simulink model "VTOLDynamics"  (R2024b)
settings: Solver=ode23t  StartTime=0.0  StopTime=10.0  FixedStep=0.001  RelTol=1e-3
undefined symbols (not defined in the file): const, contact, env, F, Flap_Activate, iniRoll, initPitch, iniYaw, Light, Limit, MIL, motorctrl, tiltIni, uavParam, uavParams, vIni, xGround, yGround, zGround
libraries: matrix_library x8, slpidlib x4, robotcorelib x4, aerolibasang x2, aerolibwind2 x2, sharedtransform x2, shared6dof x1, aerolibadyn x1, sharedutil x1, Uav_Electrical_lib x1, aerolibatmos2 x1
(part 3 of 3)

== system VTOLDynamics/Force and Moments/Aerodynamic Forces/Compute Body Frame Forces and Moments/Wind frame F& M/Lateral Channel/CY/roll factors ==
  p,q,r : Inport
  Airspeed : Inport  Port=2
  Constant : Constant  Value=uavParams.aero.CYp
      settings: AttributesFormatString=%<Value>
  Constant1 : Constant  Value=uavParams.aero.CYr
      settings: AttributesFormatString=%<Value>
  Product : Product  SaturateOnIntegerOverflow=on  OutDataTypeStr=Inherit: Same as first input
  Product1 : Product  SaturateOnIntegerOverflow=on  OutDataTypeStr=Inherit: Same as first input
  Selector : Selector  InputPortWidth=3  IndexOptions=Index vector (dialog)  Indices=[1]  OutputSizes=1
  Selector1 : Selector  InputPortWidth=3  IndexOptions=Index vector (dialog)  Indices=[3]  OutputSizes=1
  Subsystem : Subsystem
  roll rate fact : Subsystem
  CSp : Outport  VectorParamsAs1DForOutWhenUnconnected=off
  CSr : Outport  Port=2  VectorParamsAs1DForOutWhenUnconnected=off
  wires:
  Selector1/1 -> Subsystem/1(r)
  p,q,r/1 -> Selector1/1, Selector/1
  Selector/1 -> roll rate fact/1(p)
  Airspeed/1 -> Subsystem/2(Airspeed), roll rate fact/2(Airspeed)
  Subsystem/1(Yaw Rate Fac) -> Product1/2
  roll rate fact/1(Roll Rate Fac) -> Product/2
  Product1/1 -> CSr/1
  Product/1 -> CSp/1
  Constant/1 -> Product/1
  Constant1/1 -> Product1/1

== system VTOLDynamics/Force and Moments/Aerodynamic Forces/Compute Body Frame Forces and Moments/Wind frame F& M/Lateral Channel/Cl/roll factors ==
  p,q,r : Inport
  Airspeed : Inport  Port=2
  Constant : Constant  Value=uavParams.aero.Clp
      settings: AttributesFormatString=%<Value>
  Constant1 : Constant  Value=uavParams.aero.Clr
      settings: AttributesFormatString=%<Value>
  Product : Product  SaturateOnIntegerOverflow=on  OutDataTypeStr=Inherit: Same as first input
  Product1 : Product  SaturateOnIntegerOverflow=on  OutDataTypeStr=Inherit: Same as first input
  Selector : Selector  InputPortWidth=3  IndexOptions=Index vector (dialog)  Indices=[1]  OutputSizes=1
  Selector1 : Selector  InputPortWidth=3  IndexOptions=Index vector (dialog)  Indices=[3]  OutputSizes=1
  roll rate fact : Subsystem
  yaw rate fact : Subsystem
  Clp : Outport  VectorParamsAs1DForOutWhenUnconnected=off
  Clr : Outport  Port=2  VectorParamsAs1DForOutWhenUnconnected=off
  wires:
  Selector1/1 -> yaw rate fact/1(r)
  p,q,r/1 -> Selector1/1, Selector/1
  Selector/1 -> roll rate fact/1(p)
  Airspeed/1 -> roll rate fact/2(Airspeed), yaw rate fact/2(Airspeed)
  yaw rate fact/1(Yaw Rate Fac) -> Product1/2
  Constant1/1 -> Product1/1
  roll rate fact/1(Roll Rate Fac) -> Product/2
  Constant/1 -> Product/1
  Product1/1 -> Clr/1
  Product/1 -> Clp/1

== system VTOLDynamics/Force and Moments/Aerodynamic Forces/Compute Body Frame Forces and Moments/Wind frame F& M/Lateral Channel/Cn/yaw factors ==
  p,q,r : Inport
  Airspeed : Inport  Port=2
  Constant : Constant  Value=uavParams.aero.Cnp
      settings: AttributesFormatString=%<Value>
  Constant1 : Constant  Value=uavParams.aero.Cnr
      settings: AttributesFormatString=%<Value>
  Product : Product  SaturateOnIntegerOverflow=on  OutDataTypeStr=Inherit: Same as first input
  Product1 : Product  SaturateOnIntegerOverflow=on  OutDataTypeStr=Inherit: Same as first input
  Selector : Selector  InputPortWidth=3  IndexOptions=Index vector (dialog)  Indices=[3]  OutputSizes=1
  Selector1 : Selector  InputPortWidth=3  IndexOptions=Index vector (dialog)  Indices=[1]  OutputSizes=1
  roll rate fact : Subsystem
  yaw rate fact1 : Subsystem
  Cnp : Outport  VectorParamsAs1DForOutWhenUnconnected=off
  Cnr : Outport  Port=2  VectorParamsAs1DForOutWhenUnconnected=off
  wires:
  Airspeed/1 -> yaw rate fact1/2(Airspeed), roll rate fact/2(Airspeed)
  Selector/1 -> yaw rate fact1/1(r)
  p,q,r/1 -> Selector1/1, Selector/1
  Selector1/1 -> roll rate fact/1(p)
  roll rate fact/1(Roll Rate Fac) -> Product/2
  Constant/1 -> Product/1
  yaw rate fact1/1(Yaw Rate Fac) -> Product1/2
  Constant1/1 -> Product1/1
  Product1/1 -> Cnr/1
  Product/1 -> Cnp/1

== system VTOLDynamics/Force and Moments/Aerodynamic Forces/Compute Body Frame Forces and Moments/Wind frame F& M/Longitudinal Channel/CL/Lift due to pitch rate ==
  p,q,r : Inport
  Airspeed : Inport  Port=2
  Constant : Constant  Value=uavParams.aero.CLq
      settings: AttributesFormatString=%<Value>
  Product : Product  SaturateOnIntegerOverflow=on  OutDataTypeStr=Inherit: Same as first input
  Selector : Selector  InputPortWidth=3  IndexOptions=Index vector (dialog)  Indices=[2]  OutputSizes=1
  pitch rate factor : Subsystem
  CLq : Outport  VectorParamsAs1DForOutWhenUnconnected=off
  wires:
  Airspeed/1 -> pitch rate factor/2(Airspeed)
  Selector/1 -> pitch rate factor/1(q)
  p,q,r/1 -> Selector/1
  Product/1 -> CLq/1
  pitch rate factor/1(Pitch Rate Fac) -> Product/2
  Constant/1 -> Product/1

== system VTOLDynamics/Force and Moments/Aerodynamic Forces/Compute Body Frame Forces and Moments/Wind frame F& M/Longitudinal Channel/Cm/Lift due to pitch rate ==
  p,q,r : Inport
  Airspeed : Inport  Port=2
  Constant : Constant  Value=uavParams.aero.Cmq
      settings: AttributesFormatString=%<Value>
  Product : Product  SaturateOnIntegerOverflow=on  OutDataTypeStr=Inherit: Same as first input
  Selector : Selector  InputPortWidth=3  IndexOptions=Index vector (dialog)  Indices=[2]  OutputSizes=1
  pitch rate factor : Subsystem
  Cmq : Outport  VectorParamsAs1DForOutWhenUnconnected=off
  wires:
  Airspeed/1 -> pitch rate factor/2(Airspeed)
  Selector/1 -> pitch rate factor/1(q)
  p,q,r/1 -> Selector/1
  Product/1 -> Cmq/1
  pitch rate factor/1(Pitch Rate Fac) -> Product/2
  Constant/1 -> Product/1

== system VTOLDynamics/Force and Moments/Aerodynamic Forces/Compute Body Frame Forces and Moments/Wind frame F& M_original/Lateral Channel/CY/roll factors ==
  p,q,r : Inport
  Airspeed : Inport  Port=2
  Constant : Constant  Value=uavParam.aero.CYp
      settings: AttributesFormatString=%<Value>
  Constant1 : Constant  Value=uavParam.aero.CYr
      settings: AttributesFormatString=%<Value>
  Get p : Selector  InputPortWidth=3  IndexOptions=Index vector (dialog)  Indices=1  OutputSizes=[(-2)]
  Get r : Selector  InputPortWidth=3  IndexOptions=Index vector (dialog)  Indices=3  OutputSizes=[(-2)]
  Product : Product  SaturateOnIntegerOverflow=on  OutDataTypeStr=Inherit: Same as first input
  Product1 : Product  SaturateOnIntegerOverflow=on  OutDataTypeStr=Inherit: Same as first input
  Subsystem : Subsystem
  roll rate fact : Subsystem
  CYp : Outport  VectorParamsAs1DForOutWhenUnconnected=off
  CYr : Outport  Port=2  VectorParamsAs1DForOutWhenUnconnected=off
  wires:
  Get r/1 -> Subsystem/1(r)
  p,q,r/1 -> Get r/1, Get p/1
  Get p/1 -> roll rate fact/1(p)
  Airspeed/1 -> Subsystem/2(Airspeed), roll rate fact/2(Airspeed)
  Subsystem/1(Yaw Rate Fac) -> Product1/2
  Constant1/1 -> Product1/1
  roll rate fact/1(Roll Rate Fac) -> Product/2
  Constant/1 -> Product/1
  Product1/1 -> CYr/1
  Product/1 -> CYp/1

== system VTOLDynamics/Force and Moments/Aerodynamic Forces/Compute Body Frame Forces and Moments/Wind frame F& M_original/Lateral Channel/Cl/roll factors ==
  p,q,r : Inport
  Airspeed : Inport  Port=2
  Constant : Constant  Value=uavParam.aero.Clp
      settings: AttributesFormatString=%<Value>
  Constant1 : Constant  Value=uavParam.aero.Clr
      settings: AttributesFormatString=%<Value>
  Get p : Selector  InputPortWidth=3  IndexOptions=Index vector (dialog)  Indices=1  OutputSizes=[(-2)]
  Get r : Selector  InputPortWidth=3  IndexOptions=Index vector (dialog)  Indices=3  OutputSizes=[(-2)]
  Product : Product  SaturateOnIntegerOverflow=on  OutDataTypeStr=Inherit: Same as first input
  Product1 : Product  SaturateOnIntegerOverflow=on  OutDataTypeStr=Inherit: Same as first input
  roll rate fact : Subsystem
  yaw rate fact : Subsystem
  Clp : Outport  VectorParamsAs1DForOutWhenUnconnected=off
  Clr : Outport  Port=2  VectorParamsAs1DForOutWhenUnconnected=off
  wires:
  Get r/1 -> yaw rate fact/1(r)
  p,q,r/1 -> Get r/1, Get p/1
  Get p/1 -> roll rate fact/1(p)
  Airspeed/1 -> yaw rate fact/2(Airspeed), roll rate fact/2(Airspeed)
  yaw rate fact/1(Yaw Rate Fac) -> Product1/2
  Constant1/1 -> Product1/1
  roll rate fact/1(Roll Rate Fac) -> Product/2
  Constant/1 -> Product/1
  Product1/1 -> Clr/1
  Product/1 -> Clp/1

== system VTOLDynamics/Force and Moments/Aerodynamic Forces/Compute Body Frame Forces and Moments/Wind frame F& M_original/Lateral Channel/Cn/yaw factors ==
  p,q,r : Inport
  Airspeed : Inport  Port=2
  Constant : Constant  Value=uavParam.aero.Cnp
      settings: AttributesFormatString=%<Value>
  Constant1 : Constant  Value=uavParam.aero.Cnr
      settings: AttributesFormatString=%<Value>
  Get p : Selector  InputPortWidth=3  IndexOptions=Index vector (dialog)  Indices=1  OutputSizes=[(-2)]
  Get r : Selector  InputPortWidth=3  IndexOptions=Index vector (dialog)  Indices=3  OutputSizes=[(-2)]
  Product : Product  SaturateOnIntegerOverflow=on  OutDataTypeStr=Inherit: Same as first input
  Product1 : Product  SaturateOnIntegerOverflow=on  OutDataTypeStr=Inherit: Same as first input
  roll rate fact : Subsystem
  yaw rate fact1 : Subsystem
  Cnp : Outport  VectorParamsAs1DForOutWhenUnconnected=off
  Cnr : Outport  Port=2  VectorParamsAs1DForOutWhenUnconnected=off
  wires:
  Airspeed/1 -> yaw rate fact1/2(Airspeed), roll rate fact/2(Airspeed)
  Get r/1 -> yaw rate fact1/1(r)
  p,q,r/1 -> Get r/1, Get p/1
  Get p/1 -> roll rate fact/1(p)
  roll rate fact/1(Roll Rate Fac) -> Product/2
  Constant/1 -> Product/1
  yaw rate fact1/1(Yaw Rate Fac) -> Product1/2
  Constant1/1 -> Product1/1
  Product1/1 -> Cnr/1
  Product/1 -> Cnp/1

== system VTOLDynamics/Force and Moments/Aerodynamic Forces/Compute Body Frame Forces and Moments/Wind frame F& M_original/Longitudinal Channel/CL/Lift due to pitch rate ==
  p,q,r : Inport
  Airspeed : Inport  Port=2
  Constant : Constant  Value=uavParam.aero.CLq
      settings: AttributesFormatString=%<Value>
  Get q : Selector  InputPortWidth=3  IndexOptions=Index vector (dialog)  Indices=2  OutputSizes=[(-2)]
  Product : Product  SaturateOnIntegerOverflow=on  OutDataTypeStr=Inherit: Same as first input
  pitch rate factor : Subsystem
  CLq : Outport  VectorParamsAs1DForOutWhenUnconnected=off
  wires:
  Airspeed/1 -> pitch rate factor/2(Airspeed)
  Get q/1 -> pitch rate factor/1(q)
  p,q,r/1 -> Get q/1
  Product/1 -> CLq/1
  pitch rate factor/1(Pitch Rate Fac) -> Product/2
  Constant/1 -> Product/1

== system VTOLDynamics/Force and Moments/Aerodynamic Forces/Compute Body Frame Forces and Moments/Wind frame F& M_original/Longitudinal Channel/Cm/Lift due to pitch rate ==
  p,q,r : Inport
  Airspeed : Inport  Port=2
  Constant : Constant  Value=uavParam.aero.Cmq
      settings: AttributesFormatString=%<Value>
  Get q : Selector  InputPortWidth=3  IndexOptions=Index vector (dialog)  Indices=2  OutputSizes=[(-2)]
  Product : Product  SaturateOnIntegerOverflow=on  OutDataTypeStr=Inherit: Same as first input
  pitch rate factor : Subsystem
  Cmq : Outport  VectorParamsAs1DForOutWhenUnconnected=off
  wires:
  Airspeed/1 -> pitch rate factor/2(Airspeed)
  Get q/1 -> pitch rate factor/1(q)
  p,q,r/1 -> Get q/1
  Product/1 -> Cmq/1
  pitch rate factor/1(Pitch Rate Fac) -> Product/2
  Constant/1 -> Product/1

== system VTOLDynamics/Force and Moments/Aerodynamic Forces/Compute Body Frame Forces and Moments/Wind frame F& M/Lateral Channel/CY/roll factors/Subsystem ==
  r : Inport
  Airspeed : Inport  Port=2
  Cmq4 : Constant  Value=uavParams.geom.b
      settings: AttributesFormatString=%<Value>
  Gain : Gain  Gain=2
  Product1 : Product  Inputs=**/  SaturateOnIntegerOverflow=on  OutDataTypeStr=Inherit: Same as first input
  Saturation : Saturate  UpperLimit=inf  LowerLimit=0.1
      settings: AttributesFormatString="[%<LowerLimit>  %<UpperLimit>]"
  Yaw Rate Fac : Outport  VectorParamsAs1DForOutWhenUnconnected=off
  wires:
  Saturation/1 -> Gain/1
  Airspeed/1 -> Saturation/1
  Gain/1 -> Product1/3
  Product1/1 -> Yaw Rate Fac/1
  r/1 -> Product1/1
  Cmq4/1 -> Product1/2

== system VTOLDynamics/Force and Moments/Aerodynamic Forces/Compute Body Frame Forces and Moments/Wind frame F& M/Lateral Channel/CY/roll factors/roll rate fact ==
  p : Inport
  Airspeed : Inport  Port=2
  Cmq2 : Constant  Value=uavParams.geom.b
      settings: AttributesFormatString=%<Value>
  Gain : Gain  Gain=2
  Product : Product  Inputs=**/  SaturateOnIntegerOverflow=on  OutDataTypeStr=Inherit: Same as first input
  Saturation : Saturate  UpperLimit=inf  LowerLimit=0.1
      settings: AttributesFormatString="[%<LowerLimit>  %<UpperLimit>]"
  Roll Rate Fac : Outport  VectorParamsAs1DForOutWhenUnconnected=off
  wires:
  Airspeed/1 -> Saturation/1
  p/1 -> Product/1
  Product/1 -> Roll Rate Fac/1
  Saturation/1 -> Gain/1
  Cmq2/1 -> Product/2
  Gain/1 -> Product/3

== system VTOLDynamics/Force and Moments/Aerodynamic Forces/Compute Body Frame Forces and Moments/Wind frame F& M/Lateral Channel/Cl/roll factors/roll rate fact ==
  p : Inport
  Airspeed : Inport  Port=2
  Cmq2 : Constant  Value=uavParams.geom.b
      settings: AttributesFormatString=%<Value>
  Gain : Gain  Gain=2
  Product : Product  Inputs=**/  SaturateOnIntegerOverflow=on  OutDataTypeStr=Inherit: Same as first input
  Saturation : Saturate  UpperLimit=inf  LowerLimit=0.1
      settings: AttributesFormatString="[%<LowerLimit>  %<UpperLimit>]"
  Roll Rate Fac : Outport  VectorParamsAs1DForOutWhenUnconnected=off
  wires:
  Airspeed/1 -> Saturation/1
  p/1 -> Product/1
  Product/1 -> Roll Rate Fac/1
  Cmq2/1 -> Product/2
  Saturation/1 -> Gain/1
  Gain/1 -> Product/3

== system VTOLDynamics/Force and Moments/Aerodynamic Forces/Compute Body Frame Forces and Moments/Wind frame F& M/Lateral Channel/Cl/roll factors/yaw rate fact ==
  r : Inport
  Airspeed : Inport  Port=2
  Cmq4 : Constant  Value=uavParams.geom.b
      settings: AttributesFormatString=%<Value>
  Gain : Gain  Gain=2
  Product1 : Product  Inputs=**/  SaturateOnIntegerOverflow=on  OutDataTypeStr=Inherit: Same as first input
  Saturation : Saturate  UpperLimit=inf  LowerLimit=0.1
      settings: AttributesFormatString="[%<LowerLimit>  %<UpperLimit>]"
  Yaw Rate Fac : Outport
  wires:
  Airspeed/1 -> Saturation/1
  Saturation/1 -> Gain/1
  r/1 -> Product1/1
  Product1/1 -> Yaw Rate Fac/1
  Cmq4/1 -> Product1/2
  Gain/1 -> Product1/3

== system VTOLDynamics/Force and Moments/Aerodynamic Forces/Compute Body Frame Forces and Moments/Wind frame F& M/Lateral Channel/Cn/yaw factors/roll rate fact ==
  p : Inport
  Airspeed : Inport  Port=2
  Cmq2 : Constant  Value=uavParams.geom.b
      settings: AttributesFormatString=%<Value>
  Gain : Gain  Gain=2
  Product : Product  Inputs=**/  SaturateOnIntegerOverflow=on  OutDataTypeStr=Inherit: Same as first input
  Saturation : Saturate  UpperLimit=inf  LowerLimit=0.1
      settings: AttributesFormatString="[%<LowerLimit>  %<UpperLimit>]"
  Roll Rate Fac : Outport  VectorParamsAs1DForOutWhenUnconnected=off
  wires:
  Saturation/1 -> Gain/1
  Airspeed/1 -> Saturation/1
  p/1 -> Product/1
  Product/1 -> Roll Rate Fac/1
  Gain/1 -> Product/3
  Cmq2/1 -> Product/2

== system VTOLDynamics/Force and Moments/Aerodynamic Forces/Compute Body Frame Forces and Moments/Wind frame F& M/Lateral Channel/Cn/yaw factors/yaw rate fact1 ==
  r : Inport
  Airspeed : Inport  Port=2
  Cmq4 : Constant  Value=uavParams.geom.b
      settings: AttributesFormatString=%<Value>
  Gain : Gain  Gain=2
  Product1 : Product  Inputs=**/  SaturateOnIntegerOverflow=on  OutDataTypeStr=Inherit: Same as first input
  Saturation : Saturate  UpperLimit=inf  LowerLimit=0.1
      settings: AttributesFormatString="[%<LowerLimit>  %<UpperLimit>]"
  Yaw Rate Fac : Outport
  wires:
  Airspeed/1 -> Saturation/1
  Saturation/1 -> Gain/1
  r/1 -> Product1/1
  Product1/1 -> Yaw Rate Fac/1
  Cmq4/1 -> Product1/2
  Gain/1 -> Product1/3

== system VTOLDynamics/Force and Moments/Aerodynamic Forces/Compute Body Frame Forces and Moments/Wind frame F& M/Longitudinal Channel/CL/Lift due to pitch rate/pitch rate factor ==
  q : Inport
  Airspeed : Inport  Port=2
  Cmq2 : Constant  Value=uavParams.geom.c
      settings: AttributesFormatString=%<Value>
  Gain : Gain  Gain=2
  Product : Product  Inputs=**/  SaturateOnIntegerOverflow=on  OutDataTypeStr=Inherit: Same as first input
  Saturation : Saturate  UpperLimit=inf  LowerLimit=0.1
      settings: AttributesFormatString="[%<LowerLimit>  %<UpperLimit>]"
  Pitch Rate Fac : Outport  VectorParamsAs1DForOutWhenUnconnected=off
  wires:
  Cmq2/1 -> Product/2
  Airspeed/1 -> Saturation/1
  q/1 -> Product/1
  Product/1 -> Pitch Rate Fac/1
  Saturation/1 -> Gain/1
  Gain/1 -> Product/3

== system VTOLDynamics/Force and Moments/Aerodynamic Forces/Compute Body Frame Forces and Moments/Wind frame F& M/Longitudinal Channel/Cm/Lift due to pitch rate/pitch rate factor ==
  q : Inport
  Airspeed : Inport  Port=2
  Cmq2 : Constant  Value=uavParams.geom.c
      settings: AttributesFormatString=%<Value>
  Gain : Gain  Gain=2
  Product : Product  Inputs=**/  SaturateOnIntegerOverflow=on  OutDataTypeStr=Inherit: Same as first input
  Saturation : Saturate  UpperLimit=inf  LowerLimit=0.1
      settings: AttributesFormatString="[%<LowerLimit>  %<UpperLimit>]"
  Pitch Rate Fac : Outport  VectorParamsAs1DForOutWhenUnconnected=off
  wires:
  Cmq2/1 -> Product/2
  Airspeed/1 -> Saturation/1
  q/1 -> Product/1
  Product/1 -> Pitch Rate Fac/1
  Saturation/1 -> Gain/1
  Gain/1 -> Product/3

== system VTOLDynamics/Force and Moments/Aerodynamic Forces/Compute Body Frame Forces and Moments/Wind frame F& M_original/Lateral Channel/CY/roll factors/Subsystem ==
  r : Inport
  Airspeed : Inport  Port=2
  Cmq3 : Constant
      settings: AttributesFormatString=%<Value>
  Cmq4 : Constant  Value=uavParam.geom.b
      settings: AttributesFormatString=%<Value>
  Gain : Gain  Gain=2
  Product1 : Product  Inputs=***/  SaturateOnIntegerOverflow=on  OutDataTypeStr=Inherit: Same as first input
  Saturation : Saturate  UpperLimit=inf  LowerLimit=0.1
      settings: AttributesFormatString="[%<LowerLimit>  %<UpperLimit>]"
  Yaw Rate Fac : Outport  VectorParamsAs1DForOutWhenUnconnected=off
  wires:
  Saturation/1 -> Gain/1
  Cmq4/1 -> Product1/3
  Airspeed/1 -> Saturation/1
  Gain/1 -> Product1/4
  Cmq3/1 -> Product1/2
  Product1/1 -> Yaw Rate Fac/1
  r/1 -> Product1/1

== system VTOLDynamics/Force and Moments/Aerodynamic Forces/Compute Body Frame Forces and Moments/Wind frame F& M_original/Lateral Channel/CY/roll factors/roll rate fact ==
  p : Inport
  Airspeed : Inport  Port=2
  Cmq1 : Constant
      settings: AttributesFormatString=%<Value>
  Cmq2 : Constant  Value=uavParam.geom.b
      settings: AttributesFormatString=%<Value>
  Gain : Gain  Gain=2
  Product : Product  Inputs=***/  SaturateOnIntegerOverflow=on  OutDataTypeStr=Inherit: Same as first input
  Saturation : Saturate  UpperLimit=inf  LowerLimit=0.1
      settings: AttributesFormatString="[%<LowerLimit>  %<UpperLimit>]"
  Roll Rate Fac : Outport  VectorParamsAs1DForOutWhenUnconnected=off
  wires:
  Airspeed/1 -> Saturation/1
  Cmq2/1 -> Product/3
  Cmq1/1 -> Product/2
  p/1 -> Product/1
  Product/1 -> Roll Rate Fac/1
  Saturation/1 -> Gain/1
  Gain/1 -> Product/4

== system VTOLDynamics/Force and Moments/Aerodynamic Forces/Compute Body Frame Forces and Moments/Wind frame F& M_original/Lateral Channel/Cl/roll factors/roll rate fact ==
  p : Inport
  Airspeed : Inport  Port=2
  Cmq1 : Constant  Value=.5
      settings: AttributesFormatString=%<Value>
  Cmq2 : Constant  Value=uavParam.geom.b
      settings: AttributesFormatString=%<Value>
  Product : Product  Inputs=***/  SaturateOnIntegerOverflow=on  OutDataTypeStr=Inherit: Same as first input
  Saturation : Saturate  UpperLimit=inf  LowerLimit=0.1
      settings: AttributesFormatString="[%<LowerLimit>  %<UpperLimit>]"
  Roll Rate Fac : Outport  VectorParamsAs1DForOutWhenUnconnected=off
  wires:
  Saturation/1 -> Product/4
  Airspeed/1 -> Saturation/1
  Cmq2/1 -> Product/3
  Cmq1/1 -> Product/2
  p/1 -> Product/1
  Product/1 -> Roll Rate Fac/1

== system VTOLDynamics/Force and Moments/Aerodynamic Forces/Compute Body Frame Forces and Moments/Wind frame F& M_original/Lateral Channel/Cl/roll factors/yaw rate fact ==
  r : Inport
  Airspeed : Inport  Port=2
  Cmq3 : Constant  Value=.5
      settings: AttributesFormatString=%<Value>
  Cmq4 : Constant  Value=uavParam.geom.b
      settings: AttributesFormatString=%<Value>
  Product1 : Product  Inputs=***/  SaturateOnIntegerOverflow=on  OutDataTypeStr=Inherit: Same as first input
  Saturation : Saturate  UpperLimit=inf  LowerLimit=0.1
      settings: AttributesFormatString="[%<LowerLimit>  %<UpperLimit>]"
  Yaw Rate Fac : Outport
  wires:
  Airspeed/1 -> Saturation/1
  Saturation/1 -> Product1/4
  r/1 -> Product1/1
  Product1/1 -> Yaw Rate Fac/1
  Cmq4/1 -> Product1/3
  Cmq3/1 -> Product1/2

== system VTOLDynamics/Force and Moments/Aerodynamic Forces/Compute Body Frame Forces and Moments/Wind frame F& M_original/Lateral Channel/Cn/yaw factors/roll rate fact ==
  p : Inport
  Airspeed : Inport  Port=2
  Cmq1 : Constant  Value=.5
      settings: AttributesFormatString=%<Value>
  Cmq2 : Constant  Value=uavParam.geom.b
      settings: AttributesFormatString=%<Value>
  Product : Product  Inputs=***/  SaturateOnIntegerOverflow=on  OutDataTypeStr=Inherit: Same as first input
  Saturation : Saturate  UpperLimit=inf  LowerLimit=0.1
      settings: AttributesFormatString="[%<LowerLimit>  %<UpperLimit>]"
  Roll Rate Fac : Outport  VectorParamsAs1DForOutWhenUnconnected=off
  wires:
  Saturation/1 -> Product/4
  Airspeed/1 -> Saturation/1
  Cmq2/1 -> Product/3
  Cmq1/1 -> Product/2
  p/1 -> Product/1
  Product/1 -> Roll Rate Fac/1

== system VTOLDynamics/Force and Moments/Aerodynamic Forces/Compute Body Frame Forces and Moments/Wind frame F& M_original/Lateral Channel/Cn/yaw factors/yaw rate fact1 ==
  r : Inport
  Airspeed : Inport  Port=2
  Cmq3 : Constant  Value=.5
      settings: AttributesFormatString=%<Value>
  Cmq4 : Constant  Value=uavParam.geom.b
      settings: AttributesFormatString=%<Value>
  Product1 : Product  Inputs=***/  SaturateOnIntegerOverflow=on  OutDataTypeStr=Inherit: Same as first input
  Saturation : Saturate  UpperLimit=inf  LowerLimit=0.1
      settings: AttributesFormatString="[%<LowerLimit>  %<UpperLimit>]"
  Yaw Rate Fac : Outport
  wires:
  Airspeed/1 -> Saturation/1
  Saturation/1 -> Product1/4
  r/1 -> Product1/1
  Product1/1 -> Yaw Rate Fac/1
  Cmq4/1 -> Product1/3
  Cmq3/1 -> Product1/2

== system VTOLDynamics/Force and Moments/Aerodynamic Forces/Compute Body Frame Forces and Moments/Wind frame F& M_original/Longitudinal Channel/CL/Lift due to pitch rate/pitch rate factor ==
  q : Inport
  Airspeed : Inport  Port=2
  Cmq2 : Constant  Value=uavParam.geom.c
      settings: AttributesFormatString=%<Value>
  Gain : Gain  Gain=2
  Product : Product  Inputs=**/  SaturateOnIntegerOverflow=on  OutDataTypeStr=Inherit: Same as first input
  Saturation : Saturate  UpperLimit=inf  LowerLimit=0.1
      settings: AttributesFormatString="[%<LowerLimit>  %<UpperLimit>]"
  Pitch Rate Fac : Outport  VectorParamsAs1DForOutWhenUnconnected=off
  wires:
  Cmq2/1 -> Product/2
  Airspeed/1 -> Saturation/1
  q/1 -> Product/1
  Product/1 -> Pitch Rate Fac/1
  Saturation/1 -> Gain/1
  Gain/1 -> Product/3

== system VTOLDynamics/Force and Moments/Aerodynamic Forces/Compute Body Frame Forces and Moments/Wind frame F& M_original/Longitudinal Channel/Cm/Lift due to pitch rate/pitch rate factor ==
  q : Inport
  Airspeed : Inport  Port=2
  Cmq2 : Constant  Value=uavParam.geom.c
      settings: AttributesFormatString=%<Value>
  Gain : Gain  Gain=2
  Product : Product  Inputs=**/  SaturateOnIntegerOverflow=on  OutDataTypeStr=Inherit: Same as first input
  Saturation : Saturate  UpperLimit=inf  LowerLimit=0.1
      settings: AttributesFormatString="[%<LowerLimit>  %<UpperLimit>]"
  Pitch Rate Fac : Outport  VectorParamsAs1DForOutWhenUnconnected=off
  wires:
  Cmq2/1 -> Product/2
  Airspeed/1 -> Saturation/1
  q/1 -> Product/1
  Product/1 -> Pitch Rate Fac/1
  Saturation/1 -> Gain/1
  Gain/1 -> Product/3

== matlab function VTOLDynamics/Ground Truth Bus/MATLAB Function1 ==
  data: vxyz input; course output; gndSpeed output
function [course, gndSpeed] = fcn(vxyz)

vx = vxyz(1);
vy = vxyz(2);
course = atan2(vy, vx);
gndSpeed = norm([vx vy 0]);
